simulink model "ModelingContinuousSystems"  (R2025a)
settings: Solver=VariableStepAuto  StartTime=0.0  StopTime=10.0  RelTol=1e-3
undefined symbols (not defined in the file): b, k, m
settings Model: Creator=JPIRES3  LastModifiedBy=JPIRES3

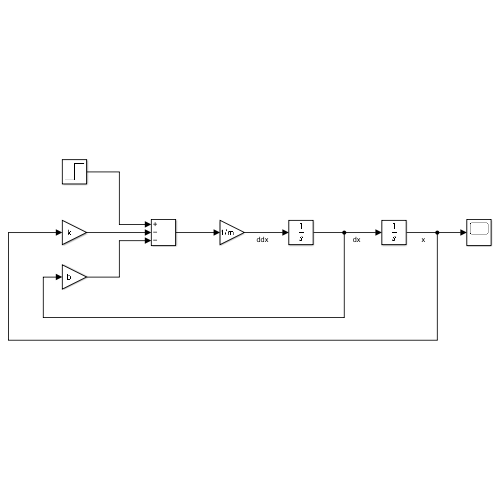
[thumbnail: Simulink's stored preview of the top-level diagram]
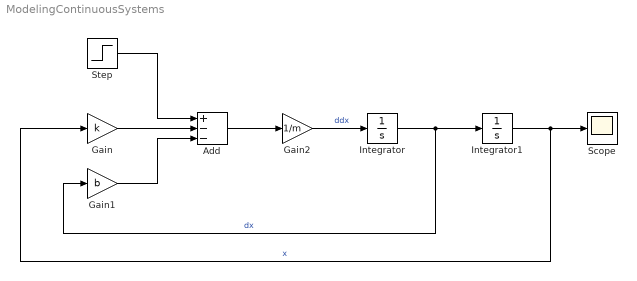
== system ModelingContinuousSystems ==
  Add : Sum  Inputs=+--
  Gain : Gain  Gain=k
  Gain1 : Gain  Gain=b
  Gain2 : Gain  Gain=1/m
  Integrator : Integrator
  Integrator1 : Integrator  InitialCondition=1
  Scope : Scope
      settings: ActiveDisplayYMinimum=-0.93011049997965212  ActiveDisplayYMaximum=1.4407088066938212
  Step : Step  After=0  SampleTime=0
  wires:
  Step/1 -> Add/1
  Gain/1 -> Add/2
  Gain1/1 -> Add/3
  Add/1 -> Gain2/1
  Gain2/1 -> Integrator/1  "ddx"
  Integrator/1 -> Gain1/1, Integrator1/1  "dx"
  Integrator1/1 -> Scope/1, Gain/1  "x"
